simulink model "eVTOL_3GL_v1"  (R2017a)
settings: Solver=VariableStepAuto  StartTime=0.0  StopTime=10.0  RelTol=1e-3
InitFcn:
  | eVTOL_3GL
values from neighbouring files (symbols this model uses):
  go = 9.80667    [eVTOL_3GL_init.m]
  k_M = f_arm/inertia    (= 0.291666666667)    [eVTOL_3GL_init.m]
  k_T = mass*go*1.8/2    (= 114.738039)    [eVTOL_3GL_init.m]
  mass = 13    [eVTOL_3GL_init.m]
  no = sqrt(mass*go/(2*k_T))    [eVTOL_3GL_init.m]
  rho = 1.24    [eVTOL_3GL_init.m]
  SCx = 0.1    [eVTOL_3GL_init.m]
  SCz = 0.3    [eVTOL_3GL_init.m]
  w_esc = 10    [eVTOL_3GL_init.m]
undefined symbols (not defined in the file or in its folder): magnitude
settings Model: Creator=augusto  LastModifiedBy=augusto
settings DataIOCC: ReturnWorkspaceOutputs=on
settings DebuggingCC: UnconnectedInputMsg=none  UnconnectedOutputMsg=none  UnconnectedLineMsg=none
settings ModelReferenceCC: EnableRefExpFcnMdlSchedulingChecks=off
settings SFSimCC: SimUseLocalCustomCode=on
settings RTWCC: RTWUseLocalCustomCode=on

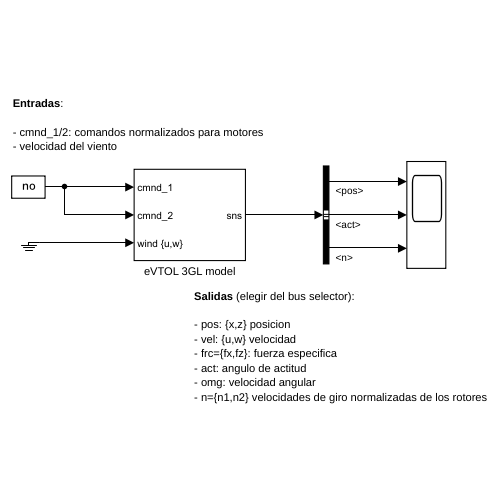
[thumbnail: Simulink's stored preview of the top-level diagram]
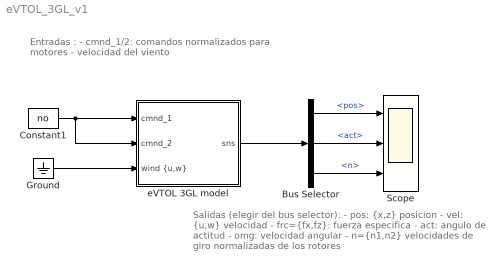
== system eVTOL_3GL_v1 ==
  note: Salidas (elegir del bus selector):
      |
      | - pos: {x,z} posicion
      | - vel: {u,w} velocidad
      | - frc={fx,fz}: fuerza especifica
      | - act: angulo de actitud
      | - omg: velocidad angular
      | - n={n1,n2} velocidades de giro normalizadas de los rotores
  note: Entradas :
      |
      | - cmnd_1/2: comandos normalizados para motores
      | - velocidad del viento
  Bus Selector : BusSelector  OutputSignals=pos,act,n
  Constant1 : Constant  Value=no
  Ground : Ground
  Scope : Scope  NumInputPorts=3
  eVTOL 3GL model : Subsystem
  wires:
  Constant1/1 -> eVTOL 3GL model/2(cmnd_2), eVTOL 3GL model/1(cmnd_1)
  eVTOL 3GL model/1(sns) -> Bus Selector/1
  Ground/1 -> eVTOL 3GL model/3("wind {u,w}")
  Bus Selector/1 -> Scope/1  "<pos>"
  Bus Selector/2 -> Scope/2  "<act>"
  Bus Selector/3 -> Scope/3  "<n>"

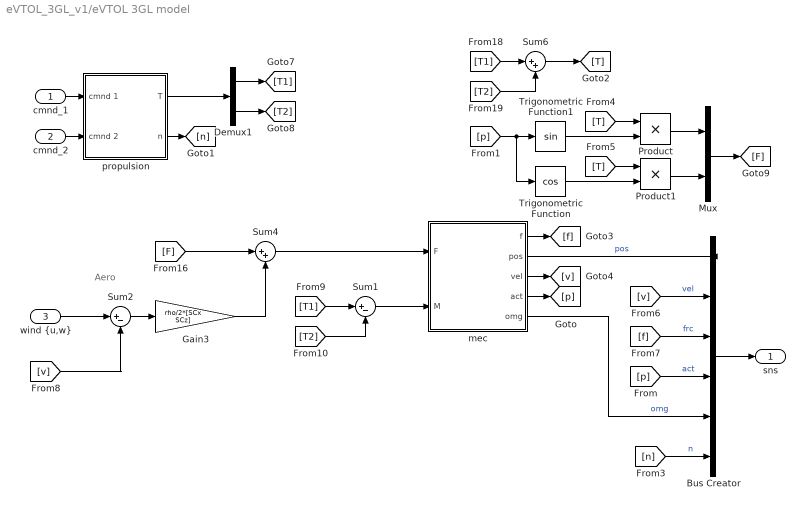
== system eVTOL_3GL_v1/eVTOL 3GL model ==
  note: Aero
  cmnd_1 : Inport
  cmnd_2 : Inport  Port=2
  "wind {u,w}" : Inport  Port=3
  Bus Creator : BusCreator  Inputs=6
  Demux1 : Demux  Outputs=2
  Gain3 : Gain  Gain=rho/2*[SCx SCz]
  Mux : Mux  Inputs=2
  Product : Product
  Product1 : Product
  Sum1 : Sum  Inputs=|+-
  Sum2 : Sum  Inputs=|+-
  Sum4 : Sum  Inputs=|++
  Sum6 : Sum  Inputs=|++
  Trigonometric Function : Trigonometry  Operator=cos
  Trigonometric Function1 : Trigonometry
  mec : Subsystem
  propulsion : Subsystem
  sns : Outport
  wires:
  [T] -> Product/1
  Trigonometric Function1/1 -> Product/2
  Bus Creator/1 -> sns/1
  [T1] -> Sum1/1
  [p] -> Bus Creator/4  "act"
  [p] -> Trigonometric Function/1, Trigonometric Function1/1
  [T] -> Product1/1
  [n] -> Bus Creator/6  "n"
  Trigonometric Function/1 -> Product1/2
  [T2] -> Sum1/2
  [f] -> Bus Creator/3  "frc"
  [F] -> Sum4/1
  Demux1/1 -> [T1]
  Demux1/2 -> [T2]
  Sum6/1 -> [T]
  [T1] -> Sum6/1
  [T2] -> Sum6/2
  Product/1 -> Mux/1
  cmnd_1/1 -> propulsion/1(cmnd 1)
  cmnd_2/1 -> propulsion/2(cmnd 2)
  propulsion/1(T) -> Demux1/1
  propulsion/2(n) -> [n]
  Gain3/1 -> Sum4/2
  Product1/1 -> Mux/2
  Mux/1 -> [F]
  Sum2/1 -> Gain3/1
  "wind {u,w}"/1 -> Sum2/1
  [v] -> Sum2/2
  [v] -> Bus Creator/2  "vel"
  Sum4/1 -> mec/1(F)
  Sum1/1 -> mec/2(M)
  mec/1(f) -> [f]
  mec/2(pos) -> Bus Creator/1  "pos"
  mec/3(vel) -> [v]
  mec/4(act) -> [p]
  mec/5(omg) -> Bus Creator/5  "omg"

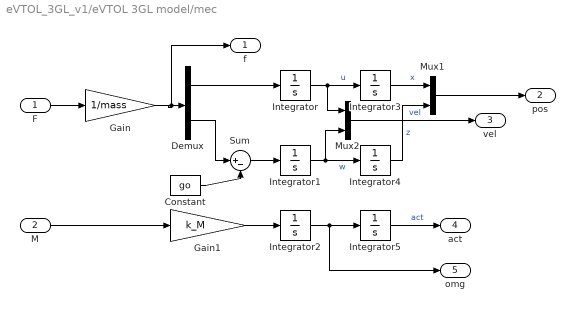
== system eVTOL_3GL_v1/eVTOL 3GL model/mec ==
  F : Inport
  M : Inport  Port=2
  Constant : Constant  Value=go
  Demux : Demux  Outputs=2
  Gain : Gain  Gain=1/mass
  Gain1 : Gain  Gain=k_M
  Integrator{,1..5} (6 alike) : Integrator
  Mux1 : Mux  Inputs=2
  Mux2 : Mux  Inputs=2
  Sum : Sum  Inputs=|+-
  f : Outport
  pos : Outport  Port=2
  vel : Outport  Port=3
  act : Outport  Port=4
  omg : Outport  Port=5
  wires:
  Constant/1 -> Sum/2
  Integrator/1 -> Mux2/1, Integrator3/1  "u"
  Gain/1 -> Demux/1, f/1
  Integrator4/1 -> Mux1/2  "z"
  Integrator2/1 -> omg/1, Integrator5/1
  Mux2/1 -> vel/1  "vel"
  Integrator1/1 -> Integrator4/1, Mux2/2  "w"
  Gain1/1 -> Integrator2/1
  Demux/2 -> Sum/1
  Integrator5/1 -> act/1  "act"
  Integrator3/1 -> Mux1/1  "x"
  F/1 -> Gain/1
  M/1 -> Gain1/1
  Mux1/1 -> pos/1
  Sum/1 -> Integrator1/1
  Demux/1 -> Integrator/1

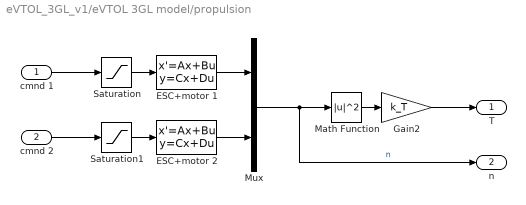
== system eVTOL_3GL_v1/eVTOL 3GL model/propulsion ==
  cmnd 1 : Inport
  cmnd 2 : Inport  Port=2
  ESC+motor 1 : StateSpace  A=-w_esc  B=w_esc  D=0  X0=no
  ESC+motor 2 : StateSpace  A=-w_esc  B=w_esc  D=0  X0=no
  Gain2 : Gain  Gain=k_T
  Math Function : Math  Operator=magnitude^2  SaturateOnIntegerOverflow=on
  Mux : Mux  Inputs=2
  Saturation : Saturate  UpperLimit=1  LowerLimit=0
  Saturation1 : Saturate  UpperLimit=1  LowerLimit=0
  T : Outport
  n : Outport  Port=2
  wires:
  ESC+motor 2/1 -> Mux/2
  Gain2/1 -> T/1
  Saturation1/1 -> ESC+motor 2/1
  cmnd 2/1 -> Saturation1/1
  Math Function/1 -> Gain2/1
  Saturation/1 -> ESC+motor 1/1
  ESC+motor 1/1 -> Mux/1
  Mux/1 -> n/1, Math Function/1  "n"
  cmnd 1/1 -> Saturation/1
